simulink model "operator"  (Simulink 8.1)
settings: Solver=ode45  StartTime=0.0  StopTime=inf  RelTol=1e-3
settings Model: Creator=eiseles  LastModifiedBy=eiseles
settings DataIOCC: SignalLoggingSaveFormat=Dataset
settings OptimizationCC: ExpressionDepthLimit=128
settings DebuggingCC: FcnCallInpInsideContextMsg=EnableAllAsError
settings GRTTargetCC: CombineOutputUpdateFcns=on  GRTInterface=off

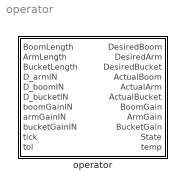
== system operator ==
  operator : Subsystem

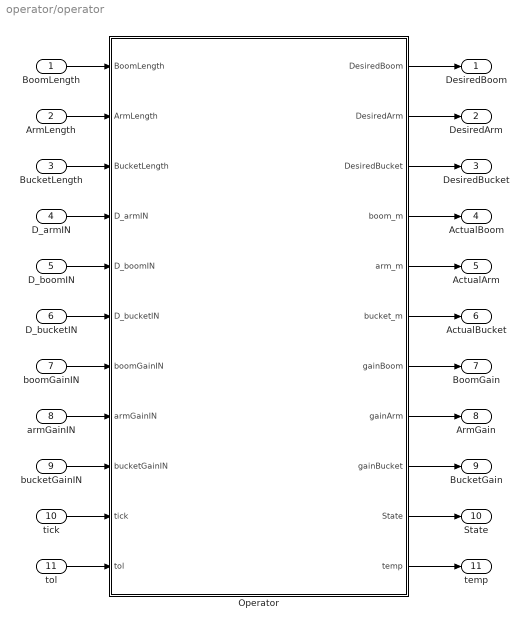
== system operator/operator ==
  BoomLength : Inport
  ArmLength : Inport  Port=2
  BucketLength : Inport  Port=3
  D_armIN : Inport  Port=4
  D_boomIN : Inport  Port=5
  D_bucketIN : Inport  Port=6
  boomGainIN : Inport  Port=7
  armGainIN : Inport  Port=8
  bucketGainIN : Inport  Port=9
  tick : Inport  Port=10
  tol : Inport  Port=11
  Operator : Stateflow chart  TreatAsAtomicUnit=on
  DesiredBoom : Outport
  DesiredArm : Outport  Port=2
  DesiredBucket : Outport  Port=3
  ActualBoom : Outport  Port=4
  ActualArm : Outport  Port=5
  ActualBucket : Outport  Port=6
  BoomGain : Outport  Port=7
  ArmGain : Outport  Port=8
  BucketGain : Outport  Port=9
  State : Outport  Port=10
  temp : Outport  Port=11
  wires:
  ArmLength/1 -> Operator/2(ArmLength)
  BoomLength/1 -> Operator/1(BoomLength)
  BucketLength/1 -> Operator/3(BucketLength)
  D_armIN/1 -> Operator/4(D_armIN)
  D_boomIN/1 -> Operator/5(D_boomIN)
  D_bucketIN/1 -> Operator/6(D_bucketIN)
  boomGainIN/1 -> Operator/7(boomGainIN)
  armGainIN/1 -> Operator/8(armGainIN)
  bucketGainIN/1 -> Operator/9(bucketGainIN)
  tick/1 -> Operator/10(tick)
  Operator/1(DesiredBoom) -> DesiredBoom/1
  Operator/2(DesiredArm) -> DesiredArm/1
  Operator/3(DesiredBucket) -> DesiredBucket/1
  Operator/4(boom_m) -> ActualBoom/1
  Operator/5(arm_m) -> ActualArm/1
  Operator/6(bucket_m) -> ActualBucket/1
  Operator/7(gainBoom) -> BoomGain/1
  Operator/8(gainArm) -> ArmGain/1
  Operator/9(gainBucket) -> BucketGain/1
  Operator/10(State) -> State/1
  Operator/11(temp) -> temp/1
  tol/1 -> Operator/11(tol)

== stateflow chart operator/Operator ==
  state intial
    en:
    temp = -1;
    State = 1;
    DesiredBoom = D_boomIN;
    DesiredArm = D_armIN;
    DesiredBucket = D_bucketIN;
    //DesiredBoom = BoomLength;
    //DesiredArm = ArmLength;
    //DesiredBucket = BucketLength;
    gainBoom = boomGainIN;
    gainArm = armGainIN;
    gainBucket = bucketGainIN;
    during:boom_m = BoomLength;
    arm_m = ArmLength;
    bucket_m = BucketLength;
  state ready
    en:
    temp = 1;
    boom_m = BoomLength;
    arm_m = ArmLength;
    bucket_m = BucketLength;
    during:boom_m = BoomLength;
    arm_m = ArmLength;
    bucket_m = BucketLength;
  state transition
    entry:
    temp = 0;
    boom_m = BoomLength;
    arm_m = ArmLength;
    bucket_m = BucketLength;
    DesiredBoom = D_boomIN;
    DesiredArm = D_armIN;
    DesiredBucket = D_bucketIN;
    during:boom_m = BoomLength;
    arm_m = ArmLength;
    bucket_m = BucketLength;
  transition -> ready : [arm_m >= DesiredArm - tol  &&...
      |  arm_m <= DesiredArm +tol  &&...
      |  boom_m >= DesiredBoom -tol &&...
      |  boom_m <= DesiredBoom +tol &&...
      |  bucket_m >= DesiredBucket -tol && ...
      |  bucket_m <= DesiredBucket + tol]
      | /State = State + 1;
  ready -> ready [order 2] : /State = 1;
  ready -> transition [order 1] : [(DesiredBoom != D_boomIN ||...
      |   DesiredArm != D_armIN ||...
      |   DesiredBucket != D_bucketIN)]
  intial -> transition : [DesiredBoom - .01 <= boom_m <= DesiredBoom +.01 &&...
      |  DesiredArm - .01    <= arm_m <= DesiredArm+.01 &&...
      |  DesiredBucket-.01 <= bucket_m <= DesiredBucket+.01]
  (default) -> intial
  data: BoomLength input double; ArmLength input double; BucketLength input double; D_armIN input double; D_boomIN input double; D_bucketIN input double; boomGainIN input double; armGainIN input double; bucketGainIN input double; tick input double; DesiredBoom output double; DesiredArm output double; DesiredBucket output double; boom_m output double; arm_m output double; bucket_m output double; gainBoom output double; gainArm output double; gainBucket output double; State output double; temp output double; tol input double
